simulink model "pwm"  (R2016b)
settings: Solver=VariableStepAuto  StartTime=0.0  StopTime=10.0  RelTol=1e-3  EnableMultiTasking=on
settings Model: Creator=Brendon  LastModifiedBy=USER
settings OptimizationCC: LifeSpan=inf
settings DebuggingCC: SFUnexpectedBacktrackingDiag=warning  SFNoUnconditionalDefaultTransitionDiag=warning  SFExecutionAtInitializationDiag=none
settings GRTTargetCC: TargetLangStandard=C89/C90 (ANSI)  GeneratePreprocessorConditionals=Disable all
settings ConfigComp: CovMetricSettings=dw  CovHtmlReporting=on  CovSaveCumulativeToWorkspaceVar=on  CovSaveSingleToWorkspaceVar=on  CovExternalEMLEnable=off

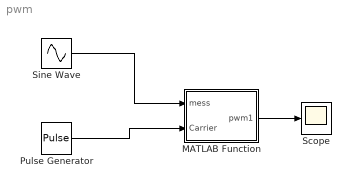
== system pwm ==
  MATLAB Function : MATLAB Function  TreatAsAtomicUnit=on
  Pulse Generator : DiscretePulseGenerator  PulseType=Time based  Period=1  PulseWidth=22
  Scope : Scope
  Sine Wave : Sin  Amplitude=5  SampleTime=0
  wires:
  Sine Wave/1 -> MATLAB Function/1(mess)
  MATLAB Function/1(pwm1) -> Scope/1
  Pulse Generator/1 -> MATLAB Function/2(Carrier)

== matlab function pwm/MATLAB Function ==
  data: mess input; pwm1 output; Carrier input
function pwm1 = pwm(mess,Carrier)

pwm1 = mess*Carrier; % the modulatation of the message and carrier
i = length(Carrier) %How long to parse for
for m = 1:i
    if(mess(m)>=Carrier(m)) %Whenever the amplitude of the message is greater than the amplitude of the carrier output a 1
        pwm1(m) = 1;
    else
        pwm1(m) = 0; %opposite from above
    end 
end
end
